simulink library "Nordic32_Lib"  (R2020b)
settings: Solver=VariableStepAuto  StartTime=0.0  StopTime=10.0  RelTol=1e-3
undefined symbols (not defined in the file or in its folder): D1, data_NREL, Delta, DiscIntNeverNeededParam, exc_Efmax, exc_Efmin, exc_Ka, exc_Ta, exc_Tb, exc_Tc, ExcData, fn, gcbh, gen_Xt, GenData, Gwind, Gwind_speed, lines, loads, mac_con, PSSData, sps_rtmsupport, time_activate_wind, trafos, wind_turbines
libraries: powerlib x18, $bdroot x13, powerlib_meascontrol x4, simulink x3, sps_avr x2, dspsigops x2, spsExcitationSystemModel x1, eeGeneralControl x1
(part 2 of 2)

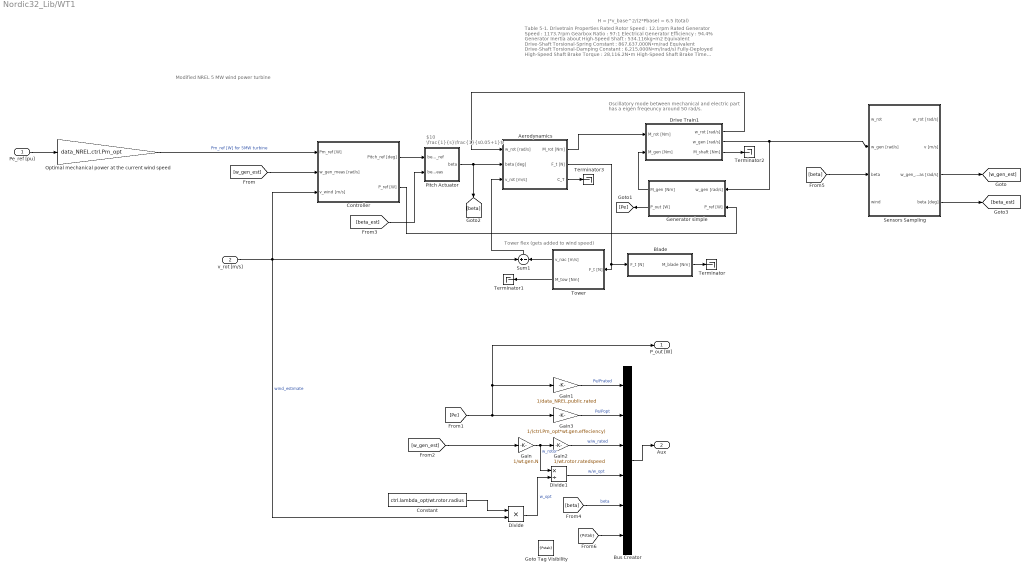
== system Nordic32_Lib/WT1 ==
  note: Oscillatory mode between mechanical and electric part has a eigen freqeuncy around 50 rad/s.
  note: $10 \frac{1}{s}\frac{1}{s0.05+1}$
  note: Tower flex (gets added to wind speed)
  note: H = J*v_base^2/(2*Pbase) = 6.5 (total)
  note: Table 5-1. Drivetrain Properties
      | Rated Rotor Speed : 12.1rpm
      | Rated Generator Speed : 1173.7rpm
      | Gearbox Ratio : 97:1
      | Electrical Generator Efficiency : 94.4%
      | Generator Inertia about High-Speed Shaft : 534.116kg•m2
      | Equivalent Drive-Shaft Torsional-Spring Constant : 867,637,000N•m/rad
      | Equivalent Drive-Shaft Torsional-Damping Constant : 6,215,000N•m/(rad/s)
      | Fully-Deployed High-Speed Shaft Brake Torque : 28,116.2N•m
      | High-Speed Shaft Brake Time Constant : 0.6s
  note: Modified NREL 5 MW wind power turbine
  Pe_ref [pu] : Inport
  v_rot [m/s] : Inport  Port=2
  Aerodynamics : Subsystem
  Blade : Subsystem
  Bus Creator : BusCreator  Inputs=6
  Constant : Constant  Value=ctrl.lambda_opt/wt.rotor.radius
  Controller : Subsystem
  Divide : Product  Inputs=**
  Divide1 : Product  Inputs=*/
  Drive Train1 : Subsystem
  Gain : Gain  Gain=1/wt.gen.N
  Gain1 : Gain  Gain=1/data_NREL.public.rated
  Gain2 : Gain  Gain=1/wt.rotor.ratedspeed
  Gain3 : Gain  Gain=1/(ctrl.Pm_opt*wt.gen.effeciency)
  Generator simple : Subsystem
  Goto Tag Visibility : GotoTagVisibility  GotoTag=Pstab
  Optimal mechanical power at the current wind speed : Gain  Gain=data_NREL.ctrl.Pm_opt
  Pitch Actuator : Subsystem
  Sensors Sampling : Subsystem
  Sum1 : Sum  Inputs=+|-  InputSameDT=on  SaturateOnIntegerOverflow=on  OutDataTypeStr=Inherit: Same as first input
  Terminator{,1..3} (4 alike) : Terminator
  "Tower " : Subsystem
  P_out [W] : Outport
  Aux : Outport  Port=2
  wires:
  Bus Creator/1 -> Aux/1
  Blade/1(M_blade [Nm]) -> Terminator/1
  Drive Train1/3(M_shaft [Nm]) -> Terminator2/1
  Generator simple/2(P_out [W]) -> [Pe]
  v_rot [m/s]/1 -> Divide/2, Controller/3(v_wind [m/s]), Sum1/1  "wind_estimate"
  Aerodynamics/2(F_t [N]) -> "Tower "/1(F_t [N]), Blade/1(F_t [N])
  Pitch Actuator/1(beta) -> [beta], Aerodynamics/2(beta [deg])
  Controller/1(Pitch_ref [deg]) -> Pitch Actuator/1(beta_ref)
  [w_gen_est] -> Gain/1
  Controller/2(P_ref [W]) -> Generator simple/2(P_ref [W])
  Generator simple/1(M_gen [Nm]) -> Drive Train1/2(M_gen [Nm])
  Drive Train1/1(w_rot [rad/s]) -> Aerodynamics/1(w_rot [rad/s])
  Aerodynamics/1(M_rot [Nm]) -> Drive Train1/1(M_rot [Nm])
  Aerodynamics/3(C_T) -> Terminator3/1
  "Tower "/1(v_nac [m/s]) -> Sum1/2
  [w_gen_est] -> Controller/2(w_gen_meas [rad/s])
  [Pe] -> Gain3/1, P_out [W]/1, Gain1/1
  Gain3/1 -> Bus Creator/2  "Pe/Popt"
  Divide1/1 -> Bus Creator/4  "w/w_opt"
  Gain1/1 -> Bus Creator/1  "Pe/Prated"
  Gain2/1 -> Bus Creator/3  "w/w_rated"
  Gain/1 -> Divide1/1, Gain2/1  "w_rotor"
  Constant/1 -> Divide/1
  Divide/1 -> Divide1/2  "w_opt"
  Optimal mechanical power at the current wind speed/1 -> Controller/1(Pm_ref [W])  "Pm_ref [W] for 5MW turbine"
  "Tower "/2(M_tow [Nm]) -> Terminator1/1
  [beta_est] -> Pitch Actuator/2(beta_meas)
  [beta] -> Bus Creator/5  "beta"
  Sum1/1 -> Aerodynamics/3(v_rot [m/s])
  Drive Train1/2(w_gen [rad/s]) -> Sensors Sampling/2(w_gen [rad/s]), Generator simple/1(w_gen [rad/s])
  [beta] -> Sensors Sampling/3(beta)
  Sensors Sampling/3(w_gen_meas [rad/s]) -> [w_gen_est]
  Sensors Sampling/4(beta [deg]) -> [beta_est]
  Pe_ref [pu]/1 -> Optimal mechanical power at the current wind speed/1
  [Pstab] -> Bus Creator/6

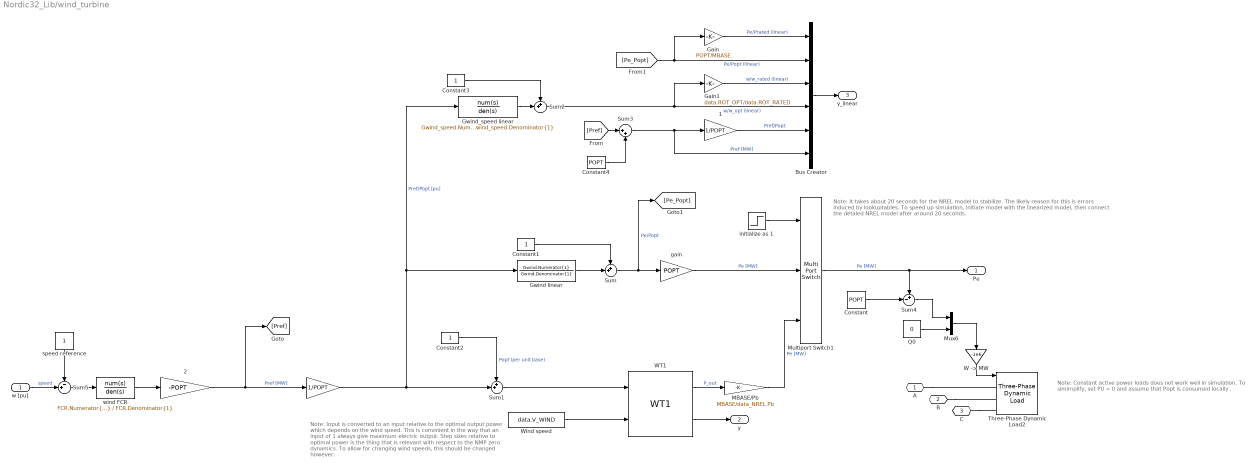
== system Nordic32_Lib/wind_turbine ==
  note: Note:
      |
      | Input is converted to an input relative to the
      | optimal output power which depends on the wind speed.
      |
      | This is convinient in the way that an input of 1 always give maximum
      | electric output. Step sizes relative to optimal power is the thing that is
      | relevant with respect to the NMP zero dynamics.
      |
      | To allow for changing wind speeds, this should be changed however.
  note: Note:
      |
      | Constant active power loads does not work well in simulation.
      | To simimplify, set P0 = 0 and assume that Popt is consumed locally .
  note: Note:
      |
      | It takes about 20 seconds for the NREL model to stabilize. The likely reason for this is errors induced by lookuptables.
      | To speed up simulation, initiate model with the linearized model, then connect the detaled NREL model after around 20 seconds.
  w [pu] : Inport
  " " : Gain  Gain=1/POPT
  " 1" : Gain  Gain=1/POPT
  " 2" : Gain  Gain=-POPT
  " gain" : Gain  Gain=POPT
  Bus Creator : BusCreator  Inputs=6
  Constant : Constant  Value=POPT
  Constant1 : Constant
  Constant2 : Constant
  Constant3 : Constant
  Constant4 : Constant  Value=POPT
  Gain : Gain  Gain=POPT/MBASE
  Gain1 : Gain  Gain=data.ROT_OPT/data.ROT_RATED
  Gwind linear : TransferFcn  Numerator=Gwind.Numerator{1}  Denominator=Gwind.Denominator{1}
  Gwind_speed linear : TransferFcn  Numerator=Gwind_speed.Numerator{1}  Denominator=Gwind_speed.Denominator{1}
  MBASE/Pb : Gain  Gain=MBASE/data_NREL.Pb
  Multiport Switch1 : MultiPortSwitch  Inputs=2  InputSameDT=on
  Mux6 : Mux  Inputs=2
  Q0 : Constant  Value=0
  Sum : Sum  Inputs=++|
  Sum1 : Sum  Inputs=++|
  Sum2 : Sum  Inputs=++|
  Sum3 : Sum  Inputs=|++
  Sum4 : Sum  Inputs=+-|
  Sum5 : Sum  Inputs=-+|
  Three-Phase Dynamic Load2 : powerlib/Elements/Three-Phase Dynamic Load  NominalVoltage=[ data.BSKV*1e3 fn ]  ActiveReactivePowers=[0 0]  PositiveSequence=[0.993047 23.2334]  ExternalControl=on  NpNq=[1.3 2]  TimeConstants="[0  0  0  0]"  MinimumVoltage=0.7  Tfilter=1e-4  LoadFlowParameters=[4,0,0,0,0]
      settings: SourceProductBaseCode=PS
  "W -> MW" : Gain  Gain=-1e6
  WT1 : $bdroot/WT1  w_gen_ini=data_NREL.w_initial  beta_ini=0  auto=off  torq_ini=data_NREL.torque_initial  data=data_NREL
  Wind speed : Constant  Value=data.V_WIND
  initialize as 1 : Step  Time=time_activate_wind  Before=1  After=2  SampleTime=0
  speed reference : Constant
  wind FCR : TransferFcn  Numerator=FCR.Numerator{1}  Denominator=FCR.Denominator{1}
  A : PMIOPort  Side=Left
  B : PMIOPort  Port=2  Side=Left
  C : PMIOPort  Port=3  Side=Left
  Pe : Outport
  y : Outport  Port=2
  y_linear : Outport  Port=3
  wires:
  Q0/1 -> Mux6/2
  w [pu]/1 -> Sum5/2  "speed"
  Mux6/1 -> "W -> MW"/1
  "W -> MW"/1 -> Three-Phase Dynamic Load2/1
  Wind speed/1 -> WT1/2
  Constant1/1 -> Sum/1
  Gwind linear/1 -> Sum/2
  Multiport Switch1/1 -> Sum4/1, Pe/1  "Pe [MW]"
  " "/1 -> Gwind_speed linear/1, Gwind linear/1, Sum1/2  "Pref/Popt [pu]"
  Constant2/1 -> Sum1/1  "Popt (per unit base)"
  WT1/2 -> y/1
  Sum1/1 -> WT1/1
  MBASE/Pb/1 -> Multiport Switch1/3  "Pe [MW]"
  initialize as 1/1 -> Multiport Switch1/1
  WT1/1 -> MBASE/Pb/1  "P_out"
  wind FCR/1 -> " 2"/1
  " gain"/1 -> Multiport Switch1/2  "Pe [MW]"
  Gain1/1 -> Bus Creator/3  "w/w_rated (linear)"
  Sum/1 -> [Pe_Popt], " gain"/1  "Pe/Popt"
  Gain/1 -> Bus Creator/1  "Pe/Prated (linear)"
  Bus Creator/1 -> y_linear/1
  Sum2/1 -> Bus Creator/4, Gain1/1  "w/w_opt (linear)"
  Constant3/1 -> Sum2/1
  Gwind_speed linear/1 -> Sum2/2
  [Pe_Popt] -> Gain/1, Bus Creator/2  "Pe/Popt (linear)"
  " 1"/1 -> Bus Creator/5  "Pref/Popt"
  Sum3/1 -> Bus Creator/6, " 1"/1  "Pref [MW]"
  Constant4/1 -> Sum3/2
  [Pref] -> Sum3/1
  Constant/1 -> Sum4/2
  Sum4/1 -> Mux6/1
  " 2"/1 -> [Pref], " "/1  "Pref [MW]"
  Sum5/1 -> wind FCR/1
  speed reference/1 -> Sum5/1
  connections:
  C/RConn1 -- Three-Phase Dynamic Load2/LConn3
  A/RConn1 -- Three-Phase Dynamic Load2/LConn1
  B/RConn1 -- Three-Phase Dynamic Load2/LConn2

== system Nordic32_Lib/Excitation/Excitation Standard ==
  Vref : Inport
  Vd : Inport  Port=2
  Vq : Inport  Port=3
  Vstab : Inport  Port=4
  Model : spsExcitationSystemModel/Continuous  tr=tr  reg=reg  exc=exc  tgr=tgr  damp=damp  sat=sat  lim=lim  v0=v0
      settings: SourceProductBaseCode=PS
  Vf : Outport  InitialOutput=0  VectorParamsAs1DForOutWhenUnconnected=off
  wires:
  Model/1 -> Vf/1
  Vref/1 -> Model/1
  Vd/1 -> Model/2
  Vq/1 -> Model/3
  Vstab/1 -> Model/4

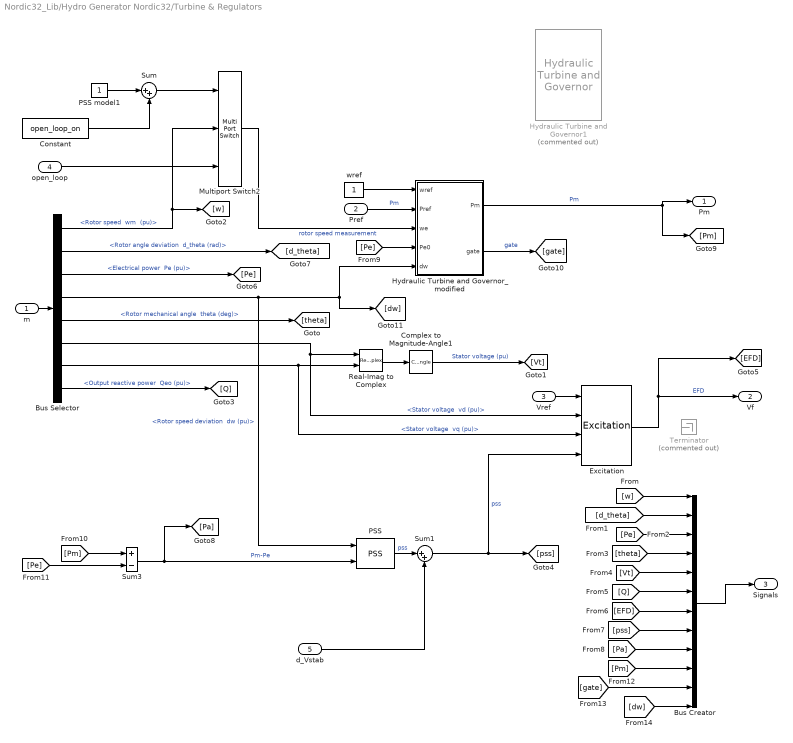
== system Nordic32_Lib/Hydro Generator Nordic32/Turbine & Regulators ==
  m : Inport
  Pref : Inport  Port=2
  Vref : Inport  Port=3
  open_loop : Inport  Port=4
  d_Vstab : Inport  Port=5
  Bus Creator : BusCreator  Inputs=12
  Bus Selector : BusSelector  OutputSignals="Mechanical.Rotor speed  wm  (pu),Mechanical.Rotor angle deviation  d_theta (rad),Mechanical.Electrical power  Pe (pu),Mechanical.Rotor speed deviation  dw (pu),Mechanical.Rotor mechanical angle  theta (deg),dq0 components.Stator voltage  vd (pu),dq0 components.Stator voltage  vq (pu),Output reactive power  Qeo (pu)"
  Complex to Magnitude-Angle1 : ComplexToMagnitudeAngle  Output=Magnitude
  Constant : Constant  Value=open_loop_on
  Excitation : $bdroot/Excitation  K_a=exc_data.K  sat_bounds=[0, 5]
  Hydraulic Turbine and Governor1 : powerlib/Machines/Hydraulic Turbine and Governor  Commented=on  sm=[ 1 gov_Ta]  gate=gov_gate  reg=gov_gain  hyd="[ 0  gov_TW]"  dref=1  po=0
      settings: SourceProductBaseCode=PS
  Hydraulic Turbine and Governor_modified : Subsystem  DialogController=POWERSYS.PowerSysDialog  mask(Hydraulic Turbine and Governor){sm=[ 1 gov_Ta], gate=gov_gate, reg=[0, 0, 0, 0, 0], hyd=[ 0  gov_TW], dref=1, po=0, gov_num=gov_num, gov_den=gov_den}
      mask prompts: sm "Servo-motor [ Ka()  Ta(sec) ]:"; gate "Gate opening limits [ gmin,gmax(pu)    vgmin,vgmax(pu/s) ]:"; reg "Permanent droop and regulator  [ Rp() Kp() Ki() Kd() Td(s) ]:"; hyd "Hydraulic turbine [ beta()  Tw(sec) ]:"; dref "Droop reference (0=power error, 1=gate opening):"; po "Initial mechanical power (pu):"
      mask help: Implements a hydraulic turbine combined with a linear FCR controller.
      mask init:
      | % block = gcb;
      | % [Ts, WantBlockChoice,ka,ta,gmin,gmax,vgmin,vgmax,Rp,Kp,ki,kd,td,beta,tw,go] = powericon('HydraulicTurbineInit',block,sm,gate,reg,hyd,po);
      | % powericon('SetInternalModels','set',block,WantBlockChoice);
      | 
      | % dialog
      | % [ Ka()  Ta(sec) ] = sm,
      | % [ gmin,gmax(pu), vgmin,vgmax(pu/s) ] =gate,
      | % [ Rp() Kp() Ki() Kd() Td(s) ] =reg,
      | %[ beta()  Tw(sec) ] = hyd
      | % Initial mechanical power (pu) = po
      | 
      | % Ts, 
      | % WantBlockChoice,
      | ka = sm(1);
      | ta = sm(2);
      | gmin = gate(1);
      | gmax = gate(2);
      | vgmin = gate(3);
      | vgmax = gate(4);
      | Rp = reg(1);
      | Kp = reg(2);
      | ki = reg(3);
      | kd = reg(4);
      | td = reg(5);
      | beta =hyd(1);
      | tw = hyd(2);
      | go = po;
      settings: OpenFcn=sps_rtmsupport('OpenFcn',gcbh)
      mask Help: helpview(psbhelp);
      mask Display: disp('')
  Multiport Switch2 : MultiPortSwitch  Inputs=2  InputSameDT=on
  "PSS " : $bdroot/PSS   Tpss=[pss_data.T1, pss_data.T2, pss_data.T3, pss_data.T4]  Kpss=pss_data.Kpss  sat_bounds=[pss_data.VMIN, pss_data.VMAX]  Tw=pss_data.Tw  Tf=pss_data.Tf
  PSS model1 : Constant
  Real-Imag to Complex : RealImagToComplex
  Sum : Sum  Inputs=|++
  Sum1 : Sum  Inputs=|++
  Sum3 : Sum  Inputs=+-  InputSameDT=on  SaturateOnIntegerOverflow=on  OutDataTypeStr=Inherit: Same as first input
  Terminator : Terminator  Commented=on
  wref : Constant
  Pm : Outport  InitialOutput=0  VectorParamsAs1DForOutWhenUnconnected=off
  Vf : Outport  Port=2  InitialOutput=0  VectorParamsAs1DForOutWhenUnconnected=off
  Signals : Outport  Port=3  InitialOutput=0  VectorParamsAs1DForOutWhenUnconnected=off
  wires:
  Bus Selector/7 -> Excitation/3, Real-Imag to Complex/2  "<Stator voltage  vq (pu)>"
  wref/1 -> Hydraulic Turbine and Governor_modified/1(wref)
  m/1 -> Bus Selector/1
  Real-Imag to Complex/1 -> Complex to Magnitude-Angle1/1
  Bus Selector/5 -> [theta]  "<Rotor mechanical angle  theta (deg)>"
  Bus Selector/6 -> Excitation/2, Real-Imag to Complex/1  "<Stator voltage  vd (pu)>"
  Bus Selector/1 -> Multiport Switch2/2, [w]  "<Rotor speed  wm  (pu)>"
  Bus Selector/2 -> [d_theta]  "<Rotor angle deviation  d_theta (rad)>"
  Bus Selector/3 -> [Pe]  "<Electrical power  Pe (pu)>"
  Bus Selector/8 -> [Q]  "<Output reactive power  Qeo (pu)>"
  Sum3/1 -> "PSS "/2, [Pa]  "Pm-Pe"
  Bus Selector/4 -> "PSS "/1, [dw], Hydraulic Turbine and Governor_modified/5(dw)  "<Rotor speed deviation  dw (pu)>"
  [w] -> Bus Creator/1
  [d_theta] -> Bus Creator/2
  [Pe] -> Bus Creator/3
  [theta] -> Bus Creator/4
  [Vt] -> Bus Creator/5
  [pss] -> Bus Creator/8
  [Pa] -> Bus Creator/9
  Bus Creator/1 -> Signals/1
  [Pe] -> Hydraulic Turbine and Governor_modified/4(Pe0)
  [Pm] -> Bus Creator/10
  Hydraulic Turbine and Governor_modified/2(gate) -> [gate]  "gate"
  [Pm] -> Sum3/1
  Complex to Magnitude-Angle1/1 -> [Vt]  "Stator voltage (pu)"
  [Q] -> Bus Creator/6
  [EFD] -> Bus Creator/7
  [Pe] -> Sum3/2
  [gate] -> Bus Creator/11
  Hydraulic Turbine and Governor_modified/1(Pm) -> Pm/1, [Pm]  "Pm"
  [dw] -> Bus Creator/12
  Pref/1 -> Hydraulic Turbine and Governor_modified/2(Pref)  "Pm"
  Vref/1 -> Excitation/1
  Excitation/1 -> Vf/1, [EFD]  "EFD"
  open_loop/1 -> Multiport Switch2/3
  Constant/1 -> Sum/2
  Sum/1 -> Multiport Switch2/1
  PSS model1/1 -> Sum/1
  Multiport Switch2/1 -> Hydraulic Turbine and Governor_modified/3(we)  "rotor speed measurement"
  Sum1/1 -> Excitation/4, [pss]  "pss"
  "PSS "/1 -> Sum1/1  "pss"
  d_Vstab/1 -> Sum1/2

== system Nordic32_Lib/Load/Local electrical freqeuncy ==
  abc : Inport
  Gain3 : Gain  Gain=1/50
  Remove initial value : $bdroot/Remove initial value  SystemSampleTime=-1  VariantActivationTime=update diagram  Latency=0  AutoFrameSizeCalculation=off
  Sequence Analyzer (Phasor)1 : powerlib_meascontrol/Measurements/Sequence Analyzer (Phasor)  seq=Positive
      settings: SourceProductBaseCode=PS
  Terminator : Terminator
  Unwrap (step size 2*pi) : $bdroot/Unwrap (step size 2*pi)  SystemSampleTime=-1  VariantActivationTime=update diagram  Latency=0  AutoFrameSizeCalculation=off
  Unwrap1 : dspsigops/Unwrap  Commented=on  tol=pi  InputProcessing=Columns as channels (frame based)  running=off
  derivative and low-pass filter : ZeroPole  Zeros=[0]  Poles=[-10 -100]  Gain=10*100
  th3 : Gain  Gain=pi/180  SaturateOnIntegerOverflow=on  OutDataTypeStr=Inherit: Same as input  ParamDataTypeStr=Inherit: Same as input
  th4 : Gain  Gain=1/(2*pi)  SaturateOnIntegerOverflow=on  OutDataTypeStr=Inherit: Same as input  ParamDataTypeStr=Inherit: Same as input
  f_local - 1 [per unit] : Outport
  wires:
  abc/1 -> Sequence Analyzer (Phasor)1/1
  Unwrap (step size 2*pi)/1 -> Remove initial value/1
  th4/1 -> Gain3/1  "f_local - 50  [Hz]"
  derivative and low-pass filter/1 -> th4/1
  Remove initial value/1 -> derivative and low-pass filter/1
  Sequence Analyzer (Phasor)1/2 -> th3/1  "deg"
  th3/1 -> Unwrap (step size 2*pi)/1  "rad"
  Gain3/1 -> f_local - 1 [per unit]/1  "f-1 [pu]"
  Sequence Analyzer (Phasor)1/1 -> Terminator/1

== system Nordic32_Lib/Remove initial value/Subsystem ==
  In1 : Inport
  Enable : EnablePort
  Out1 : Outport
  wires:
  In1/1 -> Out1/1

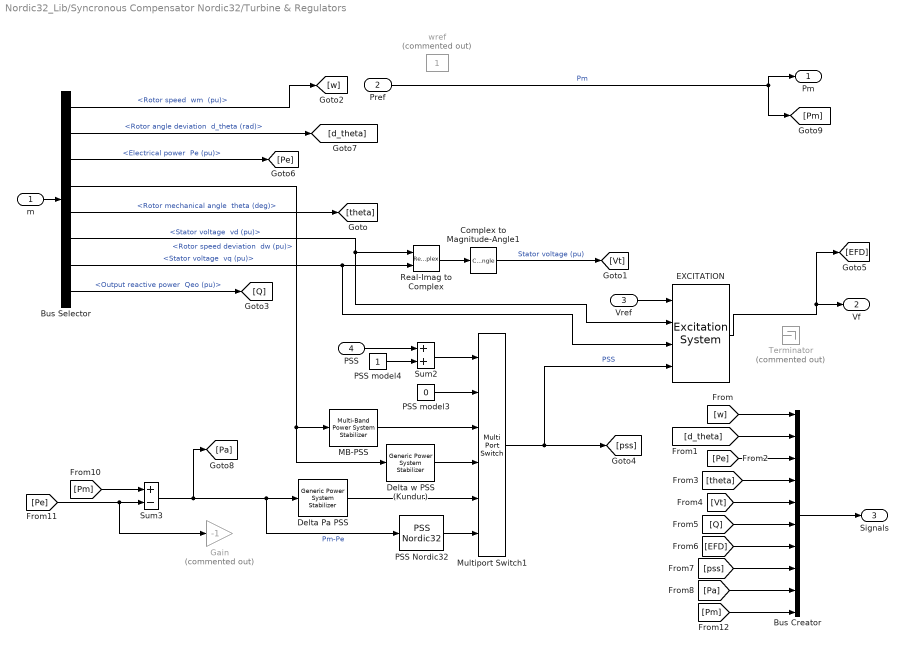
== system Nordic32_Lib/Syncronous Compensator Nordic32/Turbine & Regulators ==
  m : Inport
  Pref : Inport  Port=2
  Vref : Inport  Port=3
  PSS : Inport  Port=4
  Bus Creator : BusCreator  Inputs=10
  Bus Selector : BusSelector  OutputSignals="Mechanical.Rotor speed  wm  (pu),Mechanical.Rotor angle deviation  d_theta (rad),Mechanical.Electrical power  Pe (pu),Mechanical.Rotor speed deviation  dw (pu),Mechanical.Rotor mechanical angle  theta (deg),dq0 components.Stator voltage  vd (pu),dq0 components.Stator voltage  vq (pu),Output reactive power  Qeo (pu)"
  Complex to Magnitude-Angle1 : ComplexToMagnitudeAngle  Output=Magnitude
  "Delta Pa PSS " : powerlib/Machines/Generic Power System Stabilizer  Tsensor=15e-3  K=2.5*1.25  Twashout=1  Tleadlag1=[60e-3 1]  Tleadlag2=[0 0]  VSlimits=[-0.15 0.15]  Vinit=0  Plot_On=off  MagdB_On=on  FreqRange=logspace(-2,2,500)
      settings: SourceProductBaseCode=PS
  "Delta w PSS (Kundur) " : powerlib/Machines/Generic Power System Stabilizer  Tsensor=15e-3  K=30  Twashout=10  Tleadlag1=[50e-3 20e-3]  Tleadlag2=[3 5.4]  VSlimits=[-0.15 0.15]  Vinit=0  Plot_On=off  MagdB_On=on  FreqRange=logspace(-2,2,500)
      settings: SourceProductBaseCode=PS
  EXCITATION : sps_avr/Excitation System  tr=0  reg=[exc_Ka, exc_Ta]  exc=[ 1, 0 ]  tgr=[exc_Tb, exc_Tc]  damp=[ 1e-3 0.1]*0  sat=[ 0, 0 ]  lim=[exc_Efmin, exc_Efmax, 0 ]  v0=[1,1.07168]
      settings: SourceProductBaseCode=PS
  Gain : Gain  Commented=on  Gain=-1
  MB-PSS : powerlib/Machines/Multi-Band Power System Stabilizer  OperationMode=Simplified settings  Kg=1  GL=[0.2, 30]  GI=[1.25, 40]  GH=[12, 160]  GLd=[66 66 9.4]  TcLF=[1.667 2 0 0 0 0 2 2.4 0 0 0 0 1 1]  GId=[66 66 47.6]  TcIF=[1 1 0.25 0.3 0 0 1 1 0.3 0.36 0 0 0 0]  GHd=[66 66 233]  TcHF="[0.01 0.012 0 0 0 0  0.012 0.0144 0 0 0 0 1 1]"  LIM=[.075 .15 .15 .15]  Plot_On=off  MagdB_On=off  FreqRange=logspace(-2,2,500)
      settings: SourceProductBaseCode=PS
  Multiport Switch1 : MultiPortSwitch  Inputs=5  InputSameDT=on
  PSS Nordic32 : $bdroot/PSS  Nordic32  par=pss_data
  PSS model3 : Constant  Value=0
  PSS model4 : Constant
  Real-Imag to Complex : RealImagToComplex
  Sum2 : Sum  InputSameDT=on  SaturateOnIntegerOverflow=on  OutDataTypeStr=Inherit: Same as first input
  Sum3 : Sum  Inputs=+-  InputSameDT=on  SaturateOnIntegerOverflow=on  OutDataTypeStr=Inherit: Same as first input
  Terminator : Terminator  Commented=on
  wref : Constant  Commented=on
  Pm : Outport  InitialOutput=0  VectorParamsAs1DForOutWhenUnconnected=off
  Vf : Outport  Port=2  InitialOutput=0  VectorParamsAs1DForOutWhenUnconnected=off
  Signals : Outport  Port=3  InitialOutput=0  VectorParamsAs1DForOutWhenUnconnected=off
  wires:
  Bus Selector/7 -> EXCITATION/3, Real-Imag to Complex/2  "<Stator voltage  vq (pu)>"
  m/1 -> Bus Selector/1
  Real-Imag to Complex/1 -> Complex to Magnitude-Angle1/1
  Bus Selector/5 -> [theta]  "<Rotor mechanical angle  theta (deg)>"
  Bus Selector/6 -> Real-Imag to Complex/1, EXCITATION/2  "<Stator voltage  vd (pu)>"
  Bus Selector/1 -> [w]  "<Rotor speed  wm  (pu)>"
  Bus Selector/2 -> [d_theta]  "<Rotor angle deviation  d_theta (rad)>"
  Bus Selector/3 -> [Pe]  "<Electrical power  Pe (pu)>"
  Bus Selector/8 -> [Q]  "<Output reactive power  Qeo (pu)>"
  Sum3/1 -> [Pa], PSS Nordic32/1, "Delta Pa PSS "/1  "Pm-Pe"
  PSS/1 -> Sum2/1
  Sum2/1 -> Multiport Switch1/1
  PSS model4/1 -> Sum2/2
  "Delta Pa PSS "/1 -> Multiport Switch1/5
  "Delta w PSS (Kundur) "/1 -> Multiport Switch1/4
  MB-PSS/1 -> Multiport Switch1/3
  PSS model3/1 -> Multiport Switch1/2
  Multiport Switch1/1 -> [pss], EXCITATION/4  "PSS"
  Bus Selector/4 -> MB-PSS/1, "Delta w PSS (Kundur) "/1  "<Rotor speed deviation  dw (pu)>"
  [w] -> Bus Creator/1
  [d_theta] -> Bus Creator/2
  [Pe] -> Bus Creator/3
  [theta] -> Bus Creator/4
  [Vt] -> Bus Creator/5
  [pss] -> Bus Creator/8
  [Pa] -> Bus Creator/9
  Bus Creator/1 -> Signals/1
  [Pm] -> Bus Creator/10
  PSS Nordic32/1 -> Multiport Switch1/6
  Pref/1 -> Pm/1, [Pm]  "Pm"
  [Pm] -> Sum3/1
  Complex to Magnitude-Angle1/1 -> [Vt]  "Stator voltage (pu)"
  [Q] -> Bus Creator/6
  [EFD] -> Bus Creator/7
  [Pe] -> Gain/1, Sum3/2
  Vref/1 -> EXCITATION/1
  EXCITATION/1 -> Vf/1, [EFD]

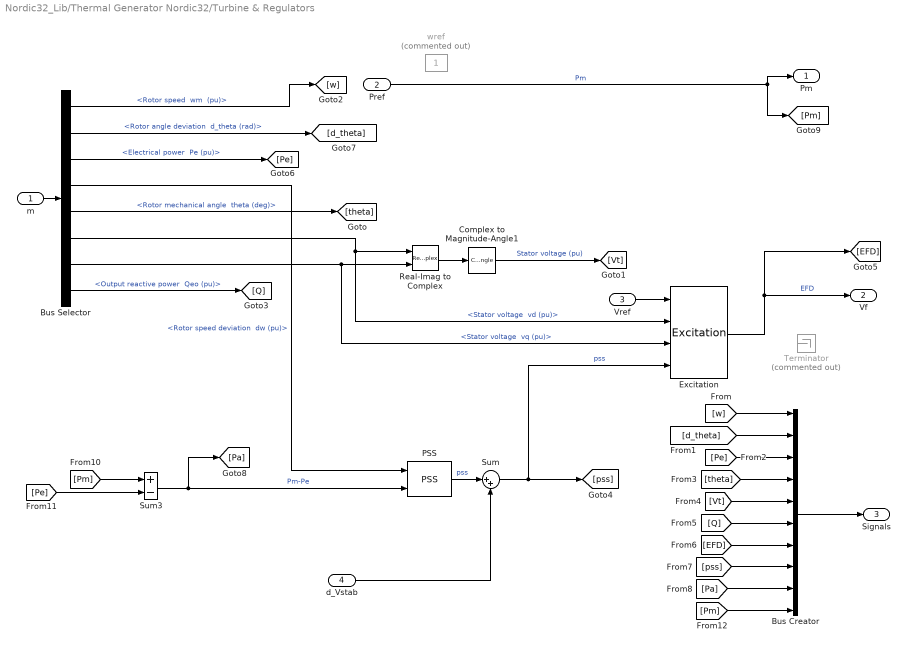
== system Nordic32_Lib/Thermal Generator Nordic32/Turbine & Regulators ==
  m : Inport
  Pref : Inport  Port=2
  Vref : Inport  Port=3
  d_Vstab : Inport  Port=4
  Bus Creator : BusCreator  Inputs=10
  Bus Selector : BusSelector  OutputSignals="Mechanical.Rotor speed  wm  (pu),Mechanical.Rotor angle deviation  d_theta (rad),Mechanical.Electrical power  Pe (pu),Mechanical.Rotor speed deviation  dw (pu),Mechanical.Rotor mechanical angle  theta (deg),dq0 components.Stator voltage  vd (pu),dq0 components.Stator voltage  vq (pu),Output reactive power  Qeo (pu)"
  Complex to Magnitude-Angle1 : ComplexToMagnitudeAngle  Output=Magnitude
  Excitation : $bdroot/Excitation  K_a=exc_data.K  sat_bounds=[0, 5]
  "PSS " : $bdroot/PSS   Tpss=[pss_data.T1, pss_data.T2, pss_data.T3, pss_data.T4]  Kpss=pss_data.Kpss  sat_bounds=[pss_data.VMIN, pss_data.VMAX]  Tw=pss_data.Tw  Tf=pss_data.Tf
  Real-Imag to Complex : RealImagToComplex
  Sum : Sum  Inputs=|++
  Sum3 : Sum  Inputs=+-  InputSameDT=on  SaturateOnIntegerOverflow=on  OutDataTypeStr=Inherit: Same as first input
  Terminator : Terminator  Commented=on
  wref : Constant  Commented=on
  Pm : Outport  InitialOutput=0  VectorParamsAs1DForOutWhenUnconnected=off
  Vf : Outport  Port=2  InitialOutput=0  VectorParamsAs1DForOutWhenUnconnected=off
  Signals : Outport  Port=3  InitialOutput=0  VectorParamsAs1DForOutWhenUnconnected=off
  wires:
  Bus Selector/7 -> Excitation/3, Real-Imag to Complex/2  "<Stator voltage  vq (pu)>"
  m/1 -> Bus Selector/1
  Real-Imag to Complex/1 -> Complex to Magnitude-Angle1/1
  Bus Selector/5 -> [theta]  "<Rotor mechanical angle  theta (deg)>"
  Bus Selector/6 -> Excitation/2, Real-Imag to Complex/1  "<Stator voltage  vd (pu)>"
  Bus Selector/1 -> [w]  "<Rotor speed  wm  (pu)>"
  Bus Selector/2 -> [d_theta]  "<Rotor angle deviation  d_theta (rad)>"
  Bus Selector/3 -> [Pe]  "<Electrical power  Pe (pu)>"
  Bus Selector/8 -> [Q]  "<Output reactive power  Qeo (pu)>"
  Sum3/1 -> "PSS "/2, [Pa]  "Pm-Pe"
  Bus Selector/4 -> "PSS "/1  "<Rotor speed deviation  dw (pu)>"
  [w] -> Bus Creator/1
  [d_theta] -> Bus Creator/2
  [Pe] -> Bus Creator/3
  [theta] -> Bus Creator/4
  [Vt] -> Bus Creator/5
  [pss] -> Bus Creator/8
  [Pa] -> Bus Creator/9
  Bus Creator/1 -> Signals/1
  [Pm] -> Bus Creator/10
  Pref/1 -> Pm/1, [Pm]  "Pm"
  [Pm] -> Sum3/1
  Complex to Magnitude-Angle1/1 -> [Vt]  "Stator voltage (pu)"
  [Q] -> Bus Creator/6
  [EFD] -> Bus Creator/7
  [Pe] -> Sum3/2
  Vref/1 -> Excitation/1
  Excitation/1 -> [EFD], Vf/1  "EFD"
  Sum/1 -> Excitation/4, [pss]  "pss"
  d_Vstab/1 -> Sum/2
  "PSS "/1 -> Sum/1  "pss"

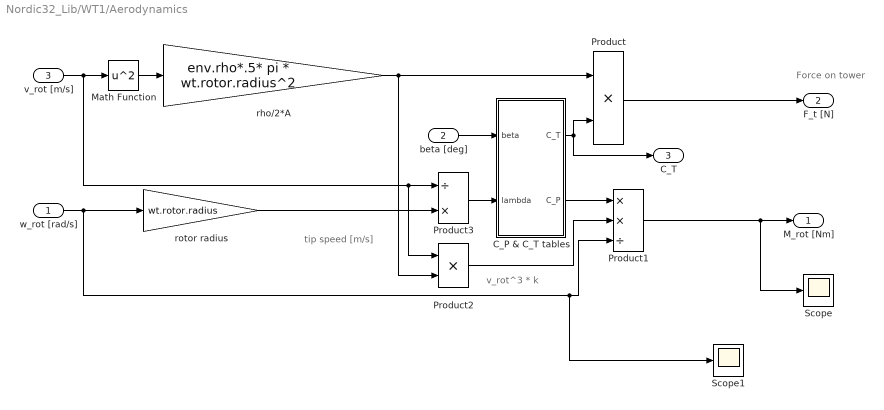
== system Nordic32_Lib/WT1/Aerodynamics ==
  note: v_rot^3 * k
  note: Force on tower
  note: tip speed
      | [m/s]
  w_rot [rad/s] : Inport
  beta [deg] : Inport  Port=2
  v_rot [m/s] : Inport  Port=3
  C_P & C_T tables : Subsystem
  Math Function : Math  Operator=square  SignedPower=on  SaturateOnIntegerOverflow=on
  Product : Product  InputSameDT=on  SaturateOnIntegerOverflow=on  OutDataTypeStr=Inherit: Same as first input
  Product1 : Product  Inputs=**/  InputSameDT=on  SaturateOnIntegerOverflow=on  OutDataTypeStr=Inherit: Same as first input
  Product2 : Product  InputSameDT=on  SaturateOnIntegerOverflow=on  OutDataTypeStr=Inherit: Same as first input
  Product3 : Product  Inputs=/*  InputSameDT=on  SaturateOnIntegerOverflow=on  OutDataTypeStr=Inherit: Same as first input
  Scope : Scope
  Scope1 : Scope
  rho/2*A : Gain  Gain=env.rho*.5* pi * wt.rotor.radius^2  SaturateOnIntegerOverflow=on  OutDataTypeStr=Inherit: Same as input  ParamDataTypeStr=Inherit: Same as input
  rotor radius : Gain  Gain=wt.rotor.radius  SaturateOnIntegerOverflow=on  OutDataTypeStr=Inherit: Same as input  ParamDataTypeStr=Inherit: Same as input
  M_rot [Nm] : Outport
  F_t [N] : Outport  Port=2
  C_T : Outport  Port=3
  wires:
  Product1/1 -> Scope/1, M_rot [Nm]/1
  Product3/1 -> C_P & C_T tables/2(lambda)
  Product2/1 -> Product1/2
  C_P & C_T tables/2(C_P) -> Product1/1
  C_P & C_T tables/1(C_T) -> Product/2, C_T/1
  beta [deg]/1 -> C_P & C_T tables/1(beta)
  Math Function/1 -> rho/2*A/1
  v_rot [m/s]/1 -> Product2/1, Product3/1, Math Function/1
  rotor radius/1 -> Product3/2
  Product/1 -> F_t [N]/1
  w_rot [rad/s]/1 -> Scope1/1, Product1/3, rotor radius/1
  rho/2*A/1 -> Product/1, Product2/2

== system Nordic32_Lib/WT1/Blade ==
  F_t [N] : Inport
  1/3*Fb*2*r : Gain  Gain=1/3*wt.rotor.radius*2  SaturateOnIntegerOverflow=on  OutDataTypeStr=Inherit: Same as input  ParamDataTypeStr=Inherit: Same as input
  M_blade [Nm] : Outport
  wires:
  F_t [N]/1 -> 1/3*Fb*2*r/1
  1/3*Fb*2*r/1 -> M_blade [Nm]/1

== system Nordic32_Lib/WT1/Controller ==
  note: $0.02\frac{s+80.8}{s+1.567} = \frac{s0.2 + 1.6}{s+1.6}$
  Pm_ref [W] : Inport
  w_gen_meas [rad/s] : Inport  Port=2
  v_wind [m/s] : Inport  Port=3
  "Measurement filter " : DiscreteStateSpace  A=wt.ctrl.alpha  B=1-wt.ctrl.alpha  C=wt.ctrl.alpha  D=1-wt.ctrl.alpha  InitialCondition=wt.ctrl.gen.ini  SampleTime=wt.ctrl.Ts
  Pitch controller : Subsystem  TreatAsAtomicUnit=on
  Product : Product  RndMeth=Zero
  Rate Limiter : RateLimiter  RisingSlewLimit=wt.ctrl.torq.ratelim  FallingSlewLimit=-wt.ctrl.torq.ratelim  SampleTimeMode=inherited  InitialCondition=wt.ctrl.torq.ini
  Rated speed : Constant  Value=wt.ctrl.gen.rated
  Region check original : Subsystem
  Sample output : ZeroOrderHold  SampleTime=wt.ctrl.Ts
  Saturation : Saturate  Commented=on  UpperLimit=wt.ctrl.torq.lim  LowerLimit=0
  Sum : Sum  Inputs=+-|
  Zero-Order Hold : ZeroOrderHold  SampleTime=wt.ctrl.Ts
  sat : Saturate  Commented=on  UpperLimit=data_NREL.wt.ctrl.p_rated  LowerLimit=0
  Pitch_ref [deg] : Outport
  P_ref [W] : Outport  Port=2
  wires:
  Region check original/2(Enable pitch controller) -> Pitch controller/Enable
  Sum/1 -> Pitch controller/1(w_gen_diff)
  Rated speed/1 -> Sum/1
  Product/1 -> Sample output/1
  Zero-Order Hold/1 -> Pitch_ref [deg]/1
  Pitch controller/1(Pitch_ref [deg]) -> Region check original/4(pitch command), Zero-Order Hold/1
  Rate Limiter/1 -> Product/2
  Region check original/1(Torque_set) -> Rate Limiter/1
  v_wind [m/s]/1 -> Region check original/3(v_wind)
  Sample output/1 -> P_ref [W]/1
  Pm_ref [W]/1 -> Pitch controller/2(P_dem), Region check original/2(Pm_ref [W])  "Pm [W] for 5MW turbine"
  w_gen_meas [rad/s]/1 -> "Measurement filter "/1  "Filtered generator speed"
  "Measurement filter "/1 -> Product/1, Region check original/1(w_gen), Sum/2  "Filtered generator speed"

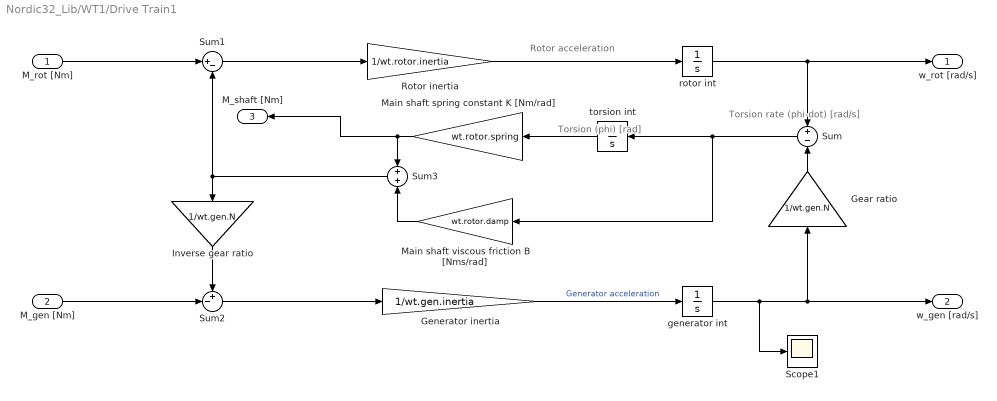
== system Nordic32_Lib/WT1/Drive Train1 ==
  note: Rotor acceleration
  note: Torsion (phi)
      | [rad]
  note: Torsion rate (phi-dot) [rad/s]
  M_rot [Nm] : Inport
  M_gen [Nm] : Inport  Port=2
  Gear ratio : Gain  Gain=1/wt.gen.N
  Generator inertia : Gain  Gain=1/wt.gen.inertia
  Inverse gear ratio : Gain  Gain=1/wt.gen.N
  Main shaft spring constant K [Nm/rad] : Gain  Gain=wt.rotor.spring
  Main shaft viscous friction B [Nms/rad] : Gain  Gain=wt.rotor.damp
  Rotor inertia : Gain  Gain=1/wt.rotor.inertia
  Scope1 : Scope
  Sum : Sum  Inputs=+|-
  Sum1 : Sum  Inputs=|+-
  Sum2 : Sum  Inputs=+-|
  Sum3 : Sum  Inputs=+|+
  generator int : Integrator  InitialCondition=wt.gen.ini
  rotor int : Integrator  InitialCondition=wt.rotor.ini
  torsion int : Integrator
  w_rot [rad/s] : Outport
  w_gen [rad/s] : Outport  Port=2
  M_shaft [Nm] : Outport  Port=3
  wires:
  Generator inertia/1 -> generator int/1  "Generator acceleration"
  Rotor inertia/1 -> rotor int/1
  Sum1/1 -> Rotor inertia/1
  Inverse gear ratio/1 -> Sum2/1
  Sum3/1 -> Sum1/2, Inverse gear ratio/1
  M_gen [Nm]/1 -> Sum2/2
  Main shaft viscous friction B [Nms/rad]/1 -> Sum3/2
  Main shaft spring constant K [Nm/rad]/1 -> M_shaft [Nm]/1, Sum3/1
  torsion int/1 -> Main shaft spring constant K [Nm/rad]/1
  Sum/1 -> Main shaft viscous friction B [Nms/rad]/1, torsion int/1
  Gear ratio/1 -> Sum/2
  generator int/1 -> Scope1/1, Gear ratio/1, w_gen [rad/s]/1
  rotor int/1 -> Sum/1, w_rot [rad/s]/1
  M_rot [Nm]/1 -> Sum1/1
  Sum2/1 -> Generator inertia/1

== system Nordic32_Lib/WT1/Generator simple ==
  note: $G(s) = \frac{10}{s + 10}$
  w_gen [rad/s] : Inport
  P_ref [W] : Inport  Port=2
  Divide : Product  Inputs=*/
  Generator Time constant : Gain  Gain=1/wt.gen.timeconstant
  Generator efficiency : Gain  Gain=wt.gen.effeciency
  Multiply : Product  Inputs=**
  Sum : Sum  Inputs=|+-
  Torque Integrator : Integrator  InitialCondition=wt.gen.torq.ini
  M_gen [Nm] : Outport
  P_out [W] : Outport  Port=2
  wires:
  Sum/1 -> Generator Time constant/1
  Generator Time constant/1 -> Torque Integrator/1
  Generator efficiency/1 -> P_out [W]/1
  Multiply/1 -> Generator efficiency/1
  Divide/1 -> Sum/1
  Torque Integrator/1 -> M_gen [Nm]/1, Multiply/1, Sum/2
  w_gen [rad/s]/1 -> Multiply/2, Divide/2
  P_ref [W]/1 -> Divide/1

== system Nordic32_Lib/WT1/Pitch Actuator ==
  beta_ref : Inport
  beta_meas : Inport  Port=2
  Pitch System : Subsystem
  Pitch controller : Subsystem
  Sum : Sum  Inputs=+-|  InputSameDT=on  SaturateOnIntegerOverflow=on  OutDataTypeStr=Inherit: Same as first input
  beta : Outport
  wires:
  beta_meas/1 -> Sum/2
  Pitch System/1(theta [deg]) -> beta/1
  beta_ref/1 -> Sum/1
  Sum/1 -> Pitch controller/1(pitch_err)
  Pitch controller/1(Uctrl) -> Pitch System/1(Upitch [V])

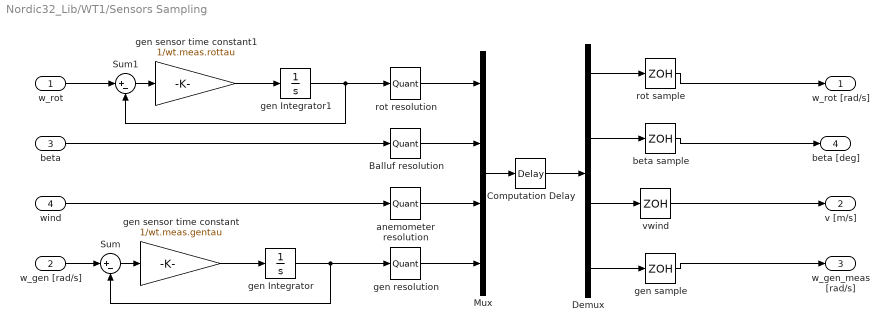
== system Nordic32_Lib/WT1/Sensors Sampling ==
  "w_rot " : Inport
  w_gen [rad/s] : Inport  Port=2
  beta : Inport  Port=3
  wind : Inport  Port=4
  Balluf resolution : Quantizer  QuantizationInterval=wt.meas.ballufres
  Computation Delay : TransportDelay  DelayTime=wt.meas.delay  InitialOutput=[wt.rotor.ini wt.pitch.ini 0 wt.gen.ini]
  Demux : Demux
  Mux : Mux
  Sum : Sum  Inputs=|+-
  Sum1 : Sum  Inputs=|+-
  anemometer resolution : Quantizer  QuantizationInterval=wt.meas.aneres
  beta sample : ZeroOrderHold  SampleTime=wt.meas.Ts
  gen Integrator : Integrator  InitialCondition=wt.gen.ini
  gen Integrator1 : Integrator  InitialCondition=wt.rotor.ini
  gen resolution : Quantizer  QuantizationInterval=wt.meas.genres
  gen sample : ZeroOrderHold  SampleTime=wt.meas.Ts
  gen sensor time constant : Gain  Gain=1/wt.meas.gentau
  gen sensor time constant1 : Gain  Gain=1/wt.meas.rottau
  rot resolution : Quantizer  QuantizationInterval=wt.meas.rotres
  rot sample : ZeroOrderHold  SampleTime=wt.meas.Ts
  vwind : ZeroOrderHold  SampleTime=wt.meas.Ts
  w_rot [rad/s] : Outport  InitialOutput=0
  v [m/s] : Outport  Port=2  InitialOutput=0
  w_gen_meas [rad/s] : Outport  Port=3  InitialOutput=0
  beta [deg] : Outport  Port=4  InitialOutput=0
  wires:
  gen resolution/1 -> Mux/4
  w_gen [rad/s]/1 -> Sum/1
  Demux/4 -> gen sample/1
  gen sample/1 -> w_gen_meas [rad/s]/1
  anemometer resolution/1 -> Mux/3
  Balluf resolution/1 -> Mux/2
  rot resolution/1 -> Mux/1
  wind/1 -> anemometer resolution/1
  Mux/1 -> Computation Delay/1
  beta/1 -> Balluf resolution/1
  Demux/1 -> rot sample/1
  rot sample/1 -> w_rot [rad/s]/1
  beta sample/1 -> beta [deg]/1
  Computation Delay/1 -> Demux/1
  Demux/2 -> beta sample/1
  Demux/3 -> vwind/1
  vwind/1 -> v [m/s]/1
  Sum/1 -> gen sensor time constant/1
  gen sensor time constant/1 -> gen Integrator/1
  gen Integrator/1 -> Sum/2, gen resolution/1
  Sum1/1 -> gen sensor time constant1/1
  gen sensor time constant1/1 -> gen Integrator1/1
  gen Integrator1/1 -> Sum1/2, rot resolution/1
  "w_rot "/1 -> Sum1/1

== system Nordic32_Lib/WT1/Tower  ==
  F_t [N] : Inport
  F_t*h : Gain  Gain=wt.tower.height  SaturateOnIntegerOverflow=on  OutDataTypeStr=Inherit: Same as input  ParamDataTypeStr=Inherit: Same as input
  Tower1 : Subsystem  mask(Tower (thrustwise)){mtop=wt.top.mass, mtow=wt.tower.mass, ftowY=wt.tower.eigfreq, dampY=wt.tower.damp}
      mask prompts: mtop "Mass of towertop [kg]"; mtow "Aequivalent tower mass [kg]"; ftowY "Tower eigenfrequency [Hz]"; dampY "Damping coefficient"
      mask help: Thrustwise dynamics of the tower
      mask init:
      | A = [-4*pi*dampY*ftowY,  -4*pi^2*ftowY^2  ; ...
      |                     1                               0       ];
      | B = [1/(mtop+mtow) ; ...
      |           0];
      | C = [1 0 ; ...
      |     0 -4*pi^2*ftowY^2*(mtop+mtow)];
      | D = zeros(2,1);
      mask Help: The thrustwise tower dynamics are modelled as a linear oscillator
  v_nac [m/s] : Outport
  M_tow [Nm] : Outport  Port=2
  wires:
  Tower1/2(F_tow [N]) -> F_t*h/1
  F_t*h/1 -> M_tow [Nm]/1
  F_t [N]/1 -> Tower1/1(FT [Nm])
  Tower1/1(vnac [m/s]) -> v_nac [m/s]/1

== system Nordic32_Lib/Hydro Generator Nordic32/Turbine & Regulators/Hydraulic Turbine and Governor_modified ==
  wref : Inport
  Pref : Inport  Port=2
  we : Inport  Port=3
  Pe0 : Inport  Port=4
  dw : Inport  Port=5
  Model : Subsystem  mask(Hydraulic Turbine and Governor){sm=sm, gate=gate, reg=reg, hyd=hyd, dref=dref, po=po}
      mask prompts: sm "Servo-motor [ Ka()  Ta(sec) ]:"; gate "Gate opening limits [ gmin,gmax(pu)    vgmin,vgmax(pu/s) ]:"; reg "Permanent droop and regulator  [ Rp() Kp() Ki() Kd() Td(s) ]:"; hyd "Hydraulic turbine [ beta()  Tw(sec) ]:"; dref "Droop reference (0=power error, 1=gate opening):"; po "Initial mechanical power (pu):"
      mask help:
      | Implements a hydraulic turbine combined with a linear FCR controller.
      |
      | 1st input: desired speed (p.u.);
      | 2nd input: desired electrical power (p.u.);
      | 3rd input: synchronous machine's actual speed (p.u., measurement output 13 of SM block);
      | 4th input: synchronous machine's actual electrical power (p.u., measurement output 14 of SM block);
      | 5th input: synchronous machine's actual speed deviation with respect to nominal (%, measurement output 15 of SM block);
      |
      | 1st output: mechanical power to be applied to the Synchronous Machine block's 1st input (p.u.);
      | 2nd output: gate opening (p.u.).
      mask init:
      | ka=sm(1);ta=sm(2);gmin=gate(1);gmax=gate(2);vgmin=gate(3);vgmax=gate(4);Rp=reg(1);kp=reg(2);ki=reg(3);kd=reg(4);td=reg(5);beta=hyd(1);tw=hyd(2);go=po*(gmax-gmin);
      mask Help: helpview(psbhelp);
  Pm : Outport  InitialOutput=0  VectorParamsAs1DForOutWhenUnconnected=off
  gate : Outport  Port=2  InitialOutput=0  VectorParamsAs1DForOutWhenUnconnected=off
  wires:
  Model/1(Pm) -> Pm/1
  Model/2(gate) -> gate/1
  dw/1 -> Model/5(dw)
  Pe0/1 -> Model/4(Pe)
  we/1 -> Model/3(we)
  Pref/1 -> Model/2(Pref)
  wref/1 -> Model/1(wref)

== system Nordic32_Lib/WT1/Aerodynamics/C_P & C_T tables ==
  beta : Inport
  lambda : Inport  Port=2
  2-D Lookup Table : Lookup_n-D  BreakpointsForDimension1=wt.ct.beta  BreakpointsForDimension2=wt.ct.tsr  IndexSearchMethod=Evenly spaced points  Table=wt.ct.table  InternalRulePriority=Speed  RndMeth=Simplest  InputSameDT=on
      settings: InputPortMap=u0,u1
  2-D Lookup Table2 : Lookup_n-D  BreakpointsForDimension1=wt.cp.beta  BreakpointsForDimension2=wt.cp.tsr  IndexSearchMethod=Evenly spaced points  Table=wt.cp.table  InternalRulePriority=Speed  RndMeth=Simplest  InputSameDT=on
      settings: InputPortMap=u0,u1
  C_T : Outport
  C_P : Outport  Port=2
  wires:
  2-D Lookup Table/1 -> C_T/1
  2-D Lookup Table2/1 -> C_P/1
  beta/1 -> 2-D Lookup Table/1, 2-D Lookup Table2/1
  lambda/1 -> 2-D Lookup Table/2, 2-D Lookup Table2/2

== system Nordic32_Lib/WT1/Controller/Pitch controller ==
  w_gen_diff : Inport
  P_dem : Inport  Port=2
  Enable : EnablePort  StatesWhenEnabling=reset  PropagateVarSize=During execution
  Discrete-Time Integrator : DiscreteIntegrator  SampleTime=wt.ctrl.Ts  LimitOutput=on  UpperSaturationLimit=wt.ctrl.pitch.ulim*pi/180  LowerSaturationLimit=wt.ctrl.pitch.llim  ICPrevOutput=DiscIntNeverNeededParam  ICPrevScaledInput=DiscIntNeverNeededParam
  Gain correction : Lookup2D  RowIndex=wt.ctrl.pitch.pwr  ColumnIndex=wt.ctrl.pitch.beta  Table=wt.ctrl.pitch.gs  LookUpMeth=Interpolation-Use End Values
  Integer Delay : Delay  DelayLength=1
  Integral gain : Gain  Gain=wt.ctrl.pitch.Igain
  Integral schedule : Product  Inputs=*/  RndMeth=Zero
  Prop schedule : Product  Inputs=*/  RndMeth=Zero
  Proportional gain : Gain  Gain=wt.ctrl.pitch.Pgain
  Rate Limiter : RateLimiter  RisingSlewLimit=wt.ctrl.pitch.ratelim  FallingSlewLimit=-wt.ctrl.pitch.ratelim  SampleTimeMode=inherited  InitialCondition=wt.ctrl.pitch.ini
  Saturation : Saturate  UpperLimit=wt.ctrl.pitch.ulim  LowerLimit=0
  Sum : Sum  Inputs=++|
  To degrees : Gain  Gain=180/pi
  Pitch_ref [deg] : Outport  OutputWhenDisabled=reset  InitialOutput=wt.ctrl.torq.beta
  wires:
  P_dem/1 -> Gain correction/1
  Integer Delay/1 -> Gain correction/2
  To degrees/1 -> Saturation/1
  w_gen_diff/1 -> Integral gain/1, Proportional gain/1
  Integral gain/1 -> Integral schedule/1
  Prop schedule/1 -> Sum/1
  Proportional gain/1 -> Prop schedule/1
  Discrete-Time Integrator/1 -> Sum/2
  Sum/1 -> To degrees/1
  Gain correction/1 -> Integral schedule/2, Prop schedule/2
  Integral schedule/1 -> Discrete-Time Integrator/1
  Rate Limiter/1 -> Integer Delay/1, Pitch_ref [deg]/1
  Saturation/1 -> Rate Limiter/1

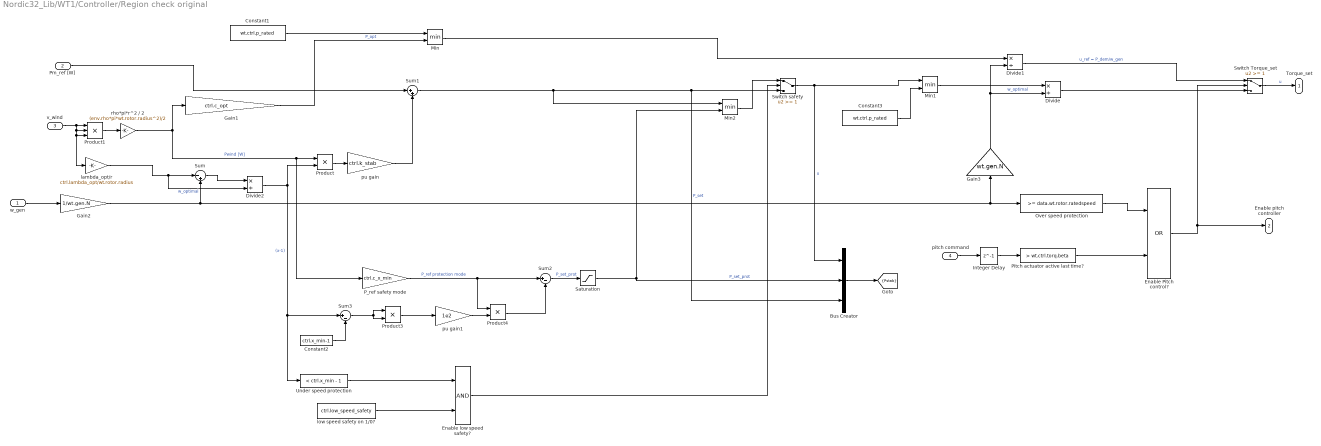
== system Nordic32_Lib/WT1/Controller/Region check original ==
  w_gen : Inport
  Pm_ref [W] : Inport  Port=2
  v_wind : Inport  Port=3
  pitch command : Inport  Port=4
  Bus Creator : BusCreator  Inputs=3
  Constant1 : Constant  Value=wt.ctrl.p_rated
  Constant2 : Constant  Value=ctrl.x_min-1
  Constant3 : Constant  Value=wt.ctrl.p_rated
  Divide : Product  Inputs=*/
  Divide1 : Product  Inputs=*/
  Divide2 : Product  Inputs=*/
  Enable Pitch control? : Logic  Operator=OR  AllPortsSameDT=off  OutDataTypeStr=boolean
  Enable low speed safety? : Logic  AllPortsSameDT=off  OutDataTypeStr=boolean
  Gain1 : Gain  Gain=ctrl.c_opt
  Gain2 : Gain  Gain=1/wt.gen.N
  Gain3 : Gain  Gain=wt.gen.N
  Integer Delay : Delay  DelayLength=1
  Min : MinMax  Inputs=2
  Min1 : MinMax  Inputs=2
  Min2 : MinMax  Inputs=2
  Over speed protection : simulink/Logic and Bit Operations/Compare To Constant  relop=>=  const=data.wt.rotor.ratedspeed  OutDataTypeStr=uint8  ZeroCross=off
  P_ref safety mode : Gain  Gain=ctrl.c_x_min
  Pitch actuator active last time? : simulink/Logic and Bit Operations/Compare To Constant  relop=>  const=wt.ctrl.torq.beta  OutDataTypeStr=uint8  ZeroCross=off
  Product : Product
  Product1 : Product  Inputs=3
  Product3 : Product
  Product4 : Product
  Saturation : Saturate  UpperLimit=wt.ctrl.p_rated  LowerLimit=0
  Sum : Sum  Inputs=|-+
  Sum1 : Sum  Inputs=|++
  Sum2 : Sum  Inputs=|+-
  Sum3 : Sum  Inputs=|+-
  Switch Torque_set : Switch  Threshold=1
  Switch safety : Switch  Threshold=1
  Under speed protection : simulink/Logic and Bit Operations/Compare To Constant  relop=<  const=ctrl.x_min - 1  OutDataTypeStr=uint8  ZeroCross=off
  lambda_opt/r : Gain  Gain=ctrl.lambda_opt/wt.rotor.radius
  low speed safety on 1/0? : Constant  Value=ctrl.low_speed_safety
  pu gain : Gain  Gain=ctrl.k_stab
  pu gain1 : Gain  Gain=1e2
  rho*pi*r^2 / 2 : Gain  Gain=(env.rho*pi*wt.rotor.radius^2)/2
  Torque_set : Outport
  Enable pitch controller : Outport  Port=2
  tag scope: Pstab=scoped
  wires:
  Enable Pitch control?/1 -> Switch Torque_set/2, Enable pitch controller/1
  Integer Delay/1 -> Pitch actuator active last time?/1
  Over speed protection/1 -> Enable Pitch control?/1
  Pitch actuator active last time?/1 -> Enable Pitch control?/2
  w_gen/1 -> Gain2/1
  pitch command/1 -> Integer Delay/1
  lambda_opt/r/1 -> Divide2/2, Sum/1  "w_optimal"
  Divide1/1 -> Switch Torque_set/1  "u_ref = P_dem/w_gen"
  v_wind/1 -> lambda_opt/r/1, Product1/3, Product1/2, Product1/1
  Product1/1 -> rho*pi*r^2 / 2/1
  Divide2/1 -> Product/2, Sum3/1, Under speed protection/1  "(x-1)"
  Product/1 -> pu gain/1
  pu gain/1 -> Sum1/2
  Pm_ref [W]/1 -> Sum1/1
  rho*pi*r^2 / 2/1 -> Gain1/1, Product/1, P_ref safety mode/1  "Pwind [W]"
  Gain1/1 -> Min/2  "P_opt"
  Switch Torque_set/1 -> Torque_set/1  "u"
  Constant1/1 -> Min/1
  Min/1 -> Divide1/1
  Sum1/1 -> Min2/1, Bus Creator/3, Switch safety/3  "P_set"
  Gain3/1 -> Divide/2, Divide1/2  "w_optimal"
  Sum/1 -> Divide2/1
  Switch safety/1 -> Bus Creator/1, Min1/1  "u"
  Enable low speed safety?/1 -> Switch safety/2
  low speed safety on 1/0?/1 -> Enable low speed safety?/2
  Under speed protection/1 -> Enable low speed safety?/1
  Min2/1 -> Switch safety/1
  P_ref safety mode/1 -> Sum2/1, Product4/1  "P_ref protection mode"
  Sum2/1 -> Saturation/1  "P_set_prot"
  Gain2/1 -> Over speed protection/1, Gain3/1, Sum/2
  Constant2/1 -> Sum3/2
  Product4/1 -> Sum2/2
  pu gain1/1 -> Product4/2
  Sum3/1 -> Product3/1, Product3/2
  Divide/1 -> Switch Torque_set/3
  Min1/1 -> Divide/1
  Constant3/1 -> Min1/2
  Bus Creator/1 -> [Pstab]
  Saturation/1 -> Bus Creator/2, Min2/2  "P_set_prot"
  Product3/1 -> pu gain1/1

== system Nordic32_Lib/WT1/Pitch Actuator/Pitch System ==
  Upitch [V] : Inport
  Hydraulic delay time : TransportDelay  DelayTime=wt.pitch.delay
  Hydraulic time constant : TransferFcn  Denominator=[wt.pitch.tau 1]
  Integrator : Integrator  InitialCondition=wt.pitch.ini
  theta [deg] : Outport
  wires:
  Hydraulic time constant/1 -> Integrator/1
  Hydraulic delay time/1 -> Hydraulic time constant/1
  Integrator/1 -> theta [deg]/1
  Upitch [V]/1 -> Hydraulic delay time/1

== system Nordic32_Lib/WT1/Pitch Actuator/Pitch controller ==
  pitch_err : Inport
  e.k : Gain  Gain=wt.pitch.K  SaturateOnIntegerOverflow=on  OutDataTypeStr=Inherit: Same as input  ParamDataTypeStr=Inherit: Same as input
  Uctrl : Outport
  wires:
  pitch_err/1 -> e.k/1
  e.k/1 -> Uctrl/1

== system Nordic32_Lib/WT1/Tower /Tower1 ==
  FT [Nm] : Inport
  Demux : Demux  Outputs=2
      settings: DisplayOption=none
  Tower : StateSpace  A=A  B=B  C=C  D=D  InitialCondition=zeros(2,1)
  vnac [m/s] : Outport  InitialOutput=0
  F_tow [N] : Outport  Port=2  InitialOutput=0
  wires:
  Demux/2 -> F_tow [N]/1
  FT [Nm]/1 -> Tower/1
  Demux/1 -> vnac [m/s]/1
  Tower/1 -> Demux/1

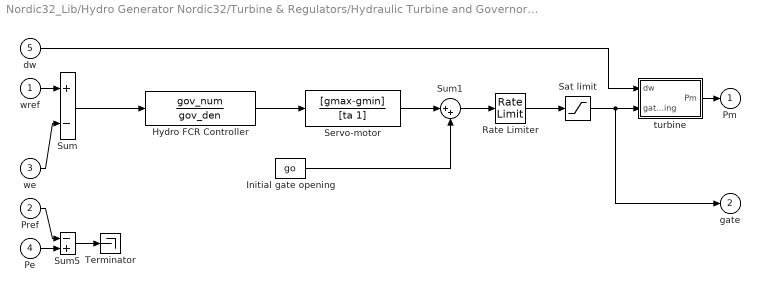
== system Nordic32_Lib/Hydro Generator Nordic32/Turbine & Regulators/Hydraulic Turbine and Governor_modified/Model ==
  wref : Inport
  Pref : Inport  Port=2
  we : Inport  Port=3
  Pe : Inport  Port=4
  dw : Inport  Port=5
  Hydro FCR Controller : TransferFcn  Numerator=gov_num  Denominator=gov_den
  Initial gate opening : Constant  Value=go
  Rate Limiter : RateLimiter  RisingSlewLimit=vgmax  FallingSlewLimit=vgmin  SampleTimeMode=inherited
  Sat limit : Saturate  UpperLimit=gmax  LowerLimit=gmin
  Servo-motor : TransferFcn  Numerator=[gmax-gmin]  Denominator=[ta 1]
  Sum : Sum  Inputs=+-  InputSameDT=on  SaturateOnIntegerOverflow=on  OutDataTypeStr=Inherit: Same as first input
  Sum1 : Sum  Inputs=|++
  Sum5 : Sum  Inputs=-+  InputSameDT=on  SaturateOnIntegerOverflow=on  OutDataTypeStr=Inherit: Same as first input
  Terminator : Terminator
  turbine : Subsystem
      mask Display: disp('hydraulic\nturbine')
  Pm : Outport  InitialOutput=0
  gate : Outport  Port=2  InitialOutput=0
  wires:
  Sat limit/1 -> gate/1, turbine/2(gate opening)
  Pe/1 -> Sum5/2
  Pref/1 -> Sum5/1
  wref/1 -> Sum/1
  we/1 -> Sum/2
  dw/1 -> turbine/1(dw)
  turbine/1(Pm) -> Pm/1
  Sum5/1 -> Terminator/1
  Sum1/1 -> Rate Limiter/1
  Hydro FCR Controller/1 -> Servo-motor/1
  Initial gate opening/1 -> Sum1/2
  Sum/1 -> Hydro FCR Controller/1
  Rate Limiter/1 -> Sat limit/1
  Servo-motor/1 -> Sum1/1

== system Nordic32_Lib/Hydro Generator Nordic32/Turbine & Regulators/Hydraulic Turbine and Governor_modified/Model/turbine ==
  dw : Inport
  gate opening : Inport  Port=2
  Constant : Constant
  Fcn : Fcn  Expr=(u(2)/u(1))^2
  Gain2 : Gain  Gain=1/tw  SaturateOnIntegerOverflow=on  OutDataTypeStr=Inherit: Same as input  ParamDataTypeStr=Inherit: Same as input
  Integrator : Integrator  InitialCondition=po
  Mux : Mux  Inputs=2
  Product : Product  InputSameDT=on  SaturateOnIntegerOverflow=on  OutDataTypeStr=Inherit: Same as first input
  Sum2 : Sum  Inputs=-+  InputSameDT=on  SaturateOnIntegerOverflow=on  OutDataTypeStr=Inherit: Same as first input
  Sum3 : Sum  Inputs=-+  InputSameDT=on  SaturateOnIntegerOverflow=on  OutDataTypeStr=Inherit: Same as first input
  beta : Gain  Gain=beta  SaturateOnIntegerOverflow=on  OutDataTypeStr=Inherit: Same as input  ParamDataTypeStr=Inherit: Same as input
  turbine gain : Gain  Gain=1/(gmax-gmin)  SaturateOnIntegerOverflow=on  OutDataTypeStr=Inherit: Same as input  ParamDataTypeStr=Inherit: Same as input
  Pm : Outport  InitialOutput=0
  wires:
  turbine gain/1 -> Mux/1
  gate opening/1 -> turbine gain/1
  Integrator/1 -> Product/2, Mux/2
  Mux/1 -> Fcn/1
  Fcn/1 -> Sum2/2
  Constant/1 -> Sum3/2
  Product/1 -> Pm/1
  Sum3/1 -> Gain2/1
  Gain2/1 -> Integrator/1
  Sum2/1 -> Sum3/1, Product/1
  beta/1 -> Sum2/1
  dw/1 -> beta/1

== matlab function Nordic32_Lib/Unwrap (step size 2*pi)/MATLAB Function ==
  data: u input; y output
function y = fcn(u)
%     u(1) = u(t)
%     u(2) = u(t-1)
%     u(3) = n    (wrap counter)

step_sensitivity = 0.5;
y = zeros(1,2);
y(2) = u(3);
if abs(u(1) - u(2)) > step_sensitivity*2*pi
    y(2) = y(2) - sign(u(1)-u(2));
end

y(1) = u(1) + y(2)*2*pi;
